simulink model "BB8_sim"  (R2015b)
settings: Solver=VariableStepAuto  StartTime=0.0  StopTime=30  RelTol=1e-3
model workspace (MAT data in the model file):
  IM = 0.0944170154667
  Il = 0.0003836
  Ke = 0.61
  Kt = 1.22
  M = 1.12
  R = 0.3556
  Ra_inv = 0.4
  g = 9.8
  l = 1.5
  r = 0.0508
libraries: simulink x3
settings Model: Creator=msearing  LastModifiedBy=zoefiddler

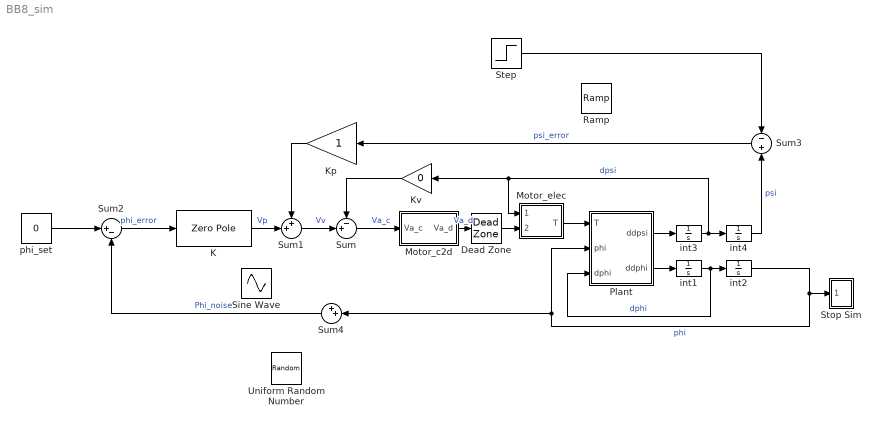
== system BB8_sim ==
  Dead Zone : DeadZone  LowerValue=-.6118  UpperValue=.6118  SaturateOnIntegerOverflow=on
  K : ZeroPole  Zeros=[-1.5]  Poles=[-0.1]  Gain=[-333]
  Kp : Gain
  Kv : Gain  Gain=0
  Motor_c2d : Subsystem
  Motor_elec : Subsystem
  Plant : Subsystem
  Ramp : simulink/Sources/Ramp  slope=10  start=1  X0=0
  Sine Wave : Sin  Amplitude=1/60  SampleTime=0
  Step : Step  After=10  SampleTime=0
  Stop Sim : Subsystem
  Sum : Sum  Inputs=-+|
  Sum1 : Sum  Inputs=++|
  Sum2 : Sum  Inputs=|+-
  Sum3 : Sum  Inputs=-|+
  Sum4 : Sum  Inputs=++|
  Uniform Random Number : UniformRandomNumber  Minimum=-1/60  Maximum=1/60  SampleTime=0.1
  int{1..4} (4 alike) : Integrator
  phi_set : Constant  Value=0
  wires:
  int4/1 -> Sum3/2  "psi"
  K/1 -> Sum1/2  "Vp"
  int2/1 -> Sum4/2, Plant/2(phi), Stop Sim/1(Phi)  "phi"
  Sum2/1 -> K/1  "phi_error"
  phi_set/1 -> Sum2/1
  Sum3/1 -> Kp/1  "psi_error"
  Kp/1 -> Sum1/1
  Sum/1 -> Motor_c2d/1(Va_c)  "Va_c"
  int1/1 -> Plant/3(dphi), int2/1  "dphi"
  int3/1 -> int4/1, Kv/1, Motor_elec/1(dpsi)  "dpsi"
  Sum1/1 -> Sum/2  "Vv"
  Kv/1 -> Sum/1
  Motor_elec/1(T) -> Plant/1(T)
  Plant/1(ddpsi) -> int3/1
  Plant/2(ddphi) -> int1/1
  Motor_c2d/1(Va_d) -> Dead Zone/1  "Va_d"
  Dead Zone/1 -> Motor_elec/2(Va_d)
  Sum4/1 -> Sum2/2  "Phi_noise"
  Step/1 -> Sum3/1

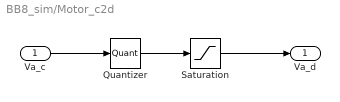
== system BB8_sim/Motor_c2d ==
  Va_c : Inport
  Quantizer : Quantizer  QuantizationInterval=12/255
  Saturation : Saturate  UpperLimit=12  LowerLimit=-12
  Va_d : Outport
  wires:
  Saturation/1 -> Va_d/1
  Va_c/1 -> Quantizer/1
  Quantizer/1 -> Saturation/1

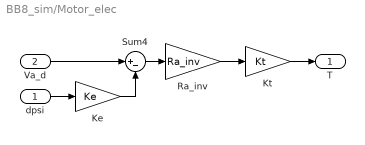
== system BB8_sim/Motor_elec ==
  dpsi : Inport
  Va_d : Inport  Port=2
  Ke : Gain  Gain=Ke
  Kt : Gain  Gain=Kt
  Ra_inv : Gain  Gain=Ra_inv
  Sum4 : Sum  Inputs=|+-
  T : Outport
  wires:
  Va_d/1 -> Sum4/1
  Sum4/1 -> Ra_inv/1
  Ke/1 -> Sum4/2
  Ra_inv/1 -> Kt/1
  dpsi/1 -> Ke/1
  Kt/1 -> T/1

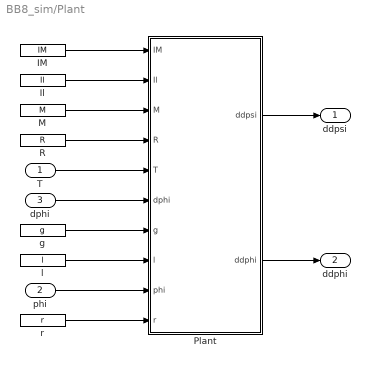
== system BB8_sim/Plant ==
  T : Inport
  phi : Inport  Port=2
  dphi : Inport  Port=3
  IM : Constant  Value=IM
  Il : Constant  Value=Il
  M : Constant  Value=M
  Plant : MATLAB Function  TreatAsAtomicUnit=on
  R : Constant  Value=R
  g : Constant  Value=g
  l : Constant  Value=l
  r : Constant  Value=r
  ddpsi : Outport
  ddphi : Outport  Port=2
  wires:
  T/1 -> Plant/5(T)
  Plant/1(ddpsi) -> ddpsi/1
  Plant/2(ddphi) -> ddphi/1
  phi/1 -> Plant/9(phi)
  dphi/1 -> Plant/6(dphi)
  IM/1 -> Plant/1(IM)
  M/1 -> Plant/3(M)
  Il/1 -> Plant/2(Il)
  r/1 -> Plant/10(r)
  l/1 -> Plant/8(l)
  g/1 -> Plant/7(g)
  R/1 -> Plant/4(R)

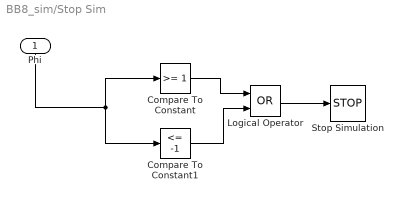
== system BB8_sim/Stop Sim ==
  Phi : Inport
  Compare To Constant : simulink/Logic and Bit Operations/Compare To Constant  relop=>=  const=1  OutDataTypeStr=boolean
  Compare To Constant1 : simulink/Logic and Bit Operations/Compare To Constant  relop=<=  const=-1  OutDataTypeStr=boolean
  Logical Operator : Logic  Operator=OR  AllPortsSameDT=off  OutDataTypeStr=boolean
  Stop Simulation : Stop
  wires:
  Compare To Constant1/1 -> Logical Operator/2
  Logical Operator/1 -> Stop Simulation/1
  Compare To Constant/1 -> Logical Operator/1
  Phi/1 -> Compare To Constant/1, Compare To Constant1/1

== matlab function BB8_sim/Plant/Plant ==
  data: IM input; Il input; M input; R input; ddpsi output; T input; dphi input; g input; l input; phi input; ddphi output; r input
function [ddpsi, ddphi] = RateFunc(IM, Il, M, R, T, dphi, g, l, phi, r)

% IM = 0;
% Il = 0;
% M = 0;
% R = 0;
% g = 0;
% l = 0;
% r = 0;
[A, b] = Eoms(IM, Il, M, R, T, dphi, g, l, phi, r);

vars = A\b;
ddphi = vars(1);
ddpsi = vars(2);
% fl = vars(3);
% nl = vars(4);
% fM = vars(5);

end
